simulink model "Noise_Shaping_ADC"  (R2012b)
settings: Solver=ode3  StartTime=0.0  StopTime=10.0  RelTol=1e-3
libraries: dspmlti4 x3, dsparch4 x1
settings Model: Creator=ayush  LastModifiedBy=ayush
settings RTWCC: RTWCompilerOptimization=On
settings ConfigurationSet: Description=SimMechanics 2G

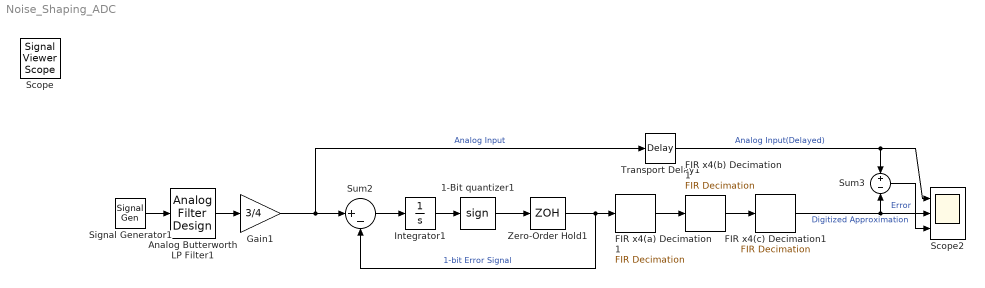
== system Noise_Shaping_ADC ==
  1-Bit quantizer1 : Signum
  Analog Butterworth LP Filter1 : dsparch4/Analog Filter Design  method=Butterworth  filttype=Lowpass  N=5  Wlo=2*pi*400  Whi=80  Rp=2  Rs=40
  FIR x4(a) Decimation1 : dspmlti4/FIR Decimation  h=fir1(31,0.15)  D=4  filtStruct=Direct form  framing=Maintain input frame size  inputOffset=0  outputBufInitCond=0  firstCoeffDataTypeStr=Inherit: Same word length as input  firstCoeffLastDataTypeStr=Inherit: Same word length as input  firstCoeffMin=[]  firstCoeffMax=[]  outputMin=[]  outputMax=[]  accumDataTypeStr=Inherit: Same as product output  accumLastDataTypeStr=Inherit: Same as product output  roundingMode=Floor  overflowMode=off  FilterSource=Specify via dialog  FilterObject=Hm_firdecim
  FIR x4(b) Decimation1 : dspmlti4/FIR Decimation  h=fir1(31,0.15)  D=4  filtStruct=Direct form  framing=Maintain input frame size  inputOffset=0  outputBufInitCond=0  firstCoeffDataTypeStr=Inherit: Same word length as input  firstCoeffLastDataTypeStr=Inherit: Same word length as input  firstCoeffMin=[]  firstCoeffMax=[]  outputMin=[]  outputMax=[]  accumDataTypeStr=Inherit: Same as product output  accumLastDataTypeStr=Inherit: Same as product output  roundingMode=Floor  overflowMode=off  FilterSource=Specify via dialog  FilterObject=Hm_firdecim
  FIR x4(c) Decimation1 : dspmlti4/FIR Decimation  h=fir1(31,0.15)  D=4  filtStruct=Direct form  framing=Maintain input frame size  inputOffset=0  outputBufInitCond=0  firstCoeffDataTypeStr=Inherit: Same word length as input  firstCoeffLastDataTypeStr=Inherit: Same word length as input  firstCoeffMin=[]  firstCoeffMax=[]  outputMin=[]  outputMax=[]  accumDataTypeStr=Inherit: Same as product output  accumLastDataTypeStr=Inherit: Same as product output  roundingMode=Floor  overflowMode=off  FilterSource=Specify via dialog  FilterObject=Hm_firdecim
  Gain1 : Gain  Gain=3/4  SaturateOnIntegerOverflow=on  OutDataTypeStr=Inherit: Same as input  ParamDataTypeStr=Inherit: Same as input
  Integrator1 : Integrator
  Scope2 : Scope  NumInputPorts=3
      settings: TimeRange=0.025  YMin=-1.1~-1.1~-0.25  YMax=1.1~1.1~0.25  MaxDataPoints=15000
  Signal Generator1 : SignalGenerator  WaveForm=square  Frequency=80
  Sum2 : Sum  Inputs=|+-  SaturateOnIntegerOverflow=on  InputSameDT=on  OutDataTypeStr=Inherit: Same as first input
  Sum3 : Sum  Inputs=+-  SaturateOnIntegerOverflow=on  InputSameDT=on  OutDataTypeStr=Inherit: Same as first input
  Transport Delay1 : TransportDelay  DelayTime=357/512000
  Zero-Order Hold1 : ZeroOrderHold  SampleTime=1/512000
  Scope : SignalViewerScope  IOType=viewer  RefreshTime=0.035000
  wires:
  Zero-Order Hold1/1 -> FIR x4(a) Decimation1/1, Sum2/2  "1-bit Error Signal"
  1-Bit quantizer1/1 -> Zero-Order Hold1/1
  Sum2/1 -> Integrator1/1
  Integrator1/1 -> 1-Bit quantizer1/1
  FIR x4(c) Decimation1/1 -> Scope2/2, Sum3/2  "Digitized Approximation"
  Gain1/1 -> Sum2/1, Transport Delay1/1  "Analog Input"
  Analog Butterworth LP Filter1/1 -> Gain1/1
  Signal Generator1/1 -> Analog Butterworth LP Filter1/1
  FIR x4(a) Decimation1/1 -> FIR x4(b) Decimation1/1
  FIR x4(b) Decimation1/1 -> FIR x4(c) Decimation1/1
  Sum3/1 -> Scope2/3  "Error"
  Transport Delay1/1 -> Sum3/1, Scope2/1  "Analog Input(Delayed)"
